simulink model "HydraTail"  (R2014b)
settings: Solver=ode3  StartTime=0.0  StopTime=inf  FixedStep=tModel  RelTol=1e-3
undefined symbols (not defined in the file or in its folder): baseGRatio, baseoffset, gcbh, rmidispblock, tipGRatio, tipoffset, tModel
libraries: legoev3lib x12, EV3Fcns x4, simulink x1
settings Model: DataDictionary=HydraTail.sldd  SimulationMode=external  ExtModeTrigDuration=2  Creator=pkaniara  LastModifiedBy=menkh
settings OptimizationCC: OptimizeModelRefInitCode=on  LifeSpan=1
settings DebuggingCC: UnderspecifiedInitializationDetection=Classic  MergeDetectMultiDrivingBlocksExec=none  SolverPrmCheckMsg=none
settings HardwareCC: ProdLargestAtomicInteger=Long  ProdLargestAtomicFloat=Float  ProdEndianess=LittleEndian  ProdHWDeviceType=ARM Compatible->ARM 9
settings RTWCC: SystemTargetFile=realtime.tlc  GenerateMakefile=off  TemplateMakefile=realtime.tmf  Description=Run on Target Hardware  RTWVerbose=off  ProcessScript=realtime_make_rtw_hook
settings STFCustomTargetCC: TargetLibSuffix=.a  GenerateSampleERTMain=on  ERTCustomFileBanners=on  SupportNonInlinedSFcns=off  SupportVariableSizeSignals=on  MATLABClassNameForMDSCustomization=Simulink.SoftwareTarget.ERTCustomization  GRTInterface=off  SystemTargetFile=realtime.tlc
settings ERTTargetCC: GenerateSampleERTMain=on  ParMdlRefBuildCompliant=off  CompOptLevelCompliant=off  ConcurrentExecutionCompliant=off  CombineOutputUpdateFcns=off  ERTFirstTimeCompliant=off  SupportContinuousTime=on  SupportVariableSizeSignals=on  ModelStepFunctionPrototypeControlCompliant=off  CPPClassGenCompliant=off  ExtMode=on  ExtModeMexArgs='192.168.10.103' 0 17725 30  InlinedParameterPlacement=NonHierarchical  ERTSrcFileBannerTemplate=realtime_code_template.cgt  ERTHdrFileBannerTemplate=realtime_code_template.cgt  ERTDataSrcFileTemplate=realtime_code_template.cgt  ERTDataHdrFileTemplate=realtime_code_template.cgt  ERTCustomFileTemplate=realtime_file_process.tlc

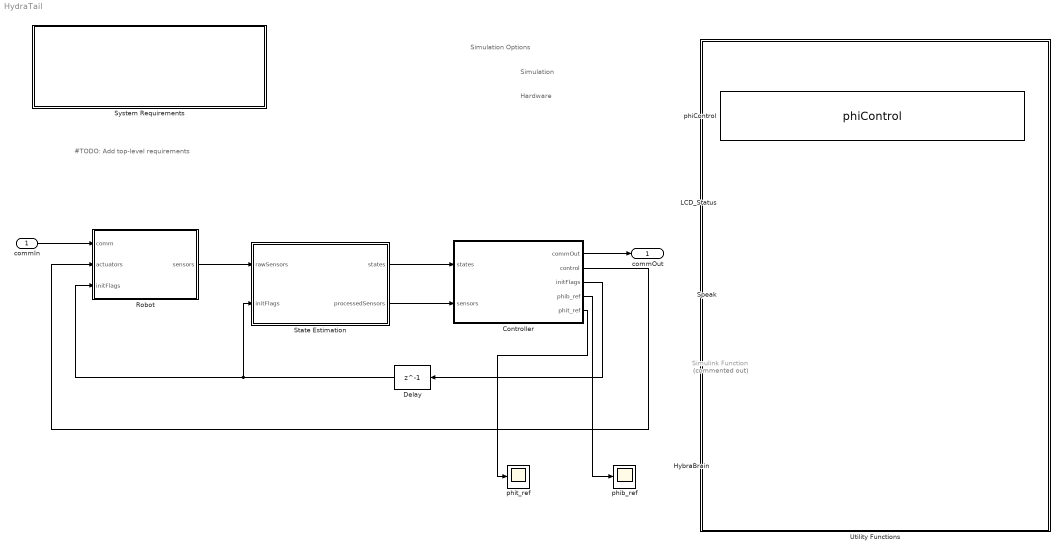
== system HydraTail ==
  note: #TODO:
      | Add top-level requirements
  note: Simulation Options
  note: Simulation
  note: Hardware
  commIn : Inport  OutDataTypeStr=Enum: Comm
  Controller : Stateflow chart  TreatAsAtomicUnit=on
  Delay : Delay  DelayLength=1  SampleTime=tModel
      settings: AttributesFormatString=Removes algebraic loop
  HybraBrain : EV3Fcns/HybraBrain
      link override 1-D Lookup Table: BreakpointsForDimension1=thetagdMod  Table=phib
      link override 1-D Lookup Table1: BreakpointsForDimension1=thetagdMod  Table=phit
  LCD_Status : EV3Fcns/LCD_Status
  Robot : Subsystem  Variant=on  VariantControl=Variant1  OverrideUsingVariant=HardwareVar
  Simulink Function : Subsystem  Commented=on  TreatAsAtomicUnit=on
  Speak : EV3Fcns/Speak
  State Estimation : Subsystem
  System Requirements : Subsystem  LoadFcn=rmidispblock('load',gcbh)  mask(System Requirements){id=SystemReq, title=System Requirements}
      mask prompts: title "Block Title"
      mask help: Lists the requirements for the current model.
      mask init:
      | id = 'SystemReq';
      | [w,h] = rmidispblock('display',gcbh);
      settings: CopyFcn=rmidispblock('create',gcbh)  DeleteFcn=rmidispblock('delete',gcbh)  ModelCloseFcn=rmidispblock('close',gcbh)  PreSaveFcn=rmidispblock('close',gcbh)  PostSaveFcn=rmidispblock('open',gcbh)  OpenFcn=rmidispblock('open',gcbh)  MoveFcn=rmidispblock('move',gcbh)
      mask Help: helpview(fullfile(docroot,'toolbox','slvnv','slvnv.map'),'systemrequirements')
      mask Display:
      | text(326/2,113-4,rmidispblock('title',gcbh),'horizontalAlignment','center','verticalAlignment','top')
      | text(w/2,h/2,'<No Requirements in System>','horizontalAlignment','center','verticalAlignment','top')
  Utility Functions : Subsystem
  phiControl : EV3Fcns/phiControl
  phib_ref : Scope
      settings: SaveName=ScopeData7
  phit_ref : Scope
      settings: SaveName=ScopeData8
  commOut : Outport  OutDataTypeStr=Enum: Comm
  wires:
  State Estimation/2(processedSensors) -> Controller/2(sensors)
  Robot/1(sensors) -> State Estimation/1(rawSensors)
  Controller/3(initFlags) -> Delay/1
  State Estimation/1(states) -> Controller/1(states)
  Delay/1 -> State Estimation/2(initFlags), Robot/3(initFlags)
  Controller/2(control) -> Robot/2(actuators)
  Controller/1(commOut) -> commOut/1
  commIn/1 -> Robot/1(comm)
  Controller/4(phib_ref) -> phib_ref/1
  Controller/5(phit_ref) -> phit_ref/1

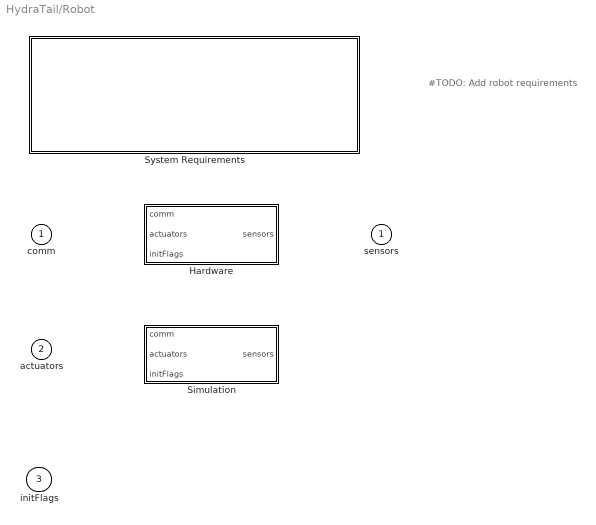
== system HydraTail/Robot ==
  note: #TODO:
      | Add robot requirements
  comm : Inport  OutDataTypeStr=Enum: Comm
  actuators : Inport  Port=2  OutDataTypeStr=Bus: ControlBus
  initFlags : Inport  Port=3  OutDataTypeStr=Bus: InitBus
  Hardware : Subsystem  VariantControl=HardwareVar
  Simulation : Subsystem  VariantControl=SimulationVar
  System Requirements : Subsystem  LoadFcn=rmidispblock('load',gcbh)  VariantControl=Variant  mask(System Requirements){id=SystemReq, title=System Requirements}
      mask prompts: title "Block Title"
      mask help: Lists the requirements for the current model.
      mask init:
      | id = 'SystemReq';
      | [w,h] = rmidispblock('display',gcbh);
      settings: CopyFcn=rmidispblock('create',gcbh)  DeleteFcn=rmidispblock('delete',gcbh)  ModelCloseFcn=rmidispblock('close',gcbh)  PreSaveFcn=rmidispblock('close',gcbh)  PostSaveFcn=rmidispblock('open',gcbh)  OpenFcn=rmidispblock('open',gcbh)  MoveFcn=rmidispblock('move',gcbh)
      mask Help: helpview(fullfile(docroot,'toolbox','slvnv','slvnv.map'),'systemrequirements')
      mask Display:
      | text(326/2,113-4,rmidispblock('title',gcbh),'horizontalAlignment','center','verticalAlignment','top')
      | text(w/2,h/2,'<No Requirements in System>','horizontalAlignment','center','verticalAlignment','top')
  sensors : Outport  OutDataTypeStr=Bus: Sensors_Bus

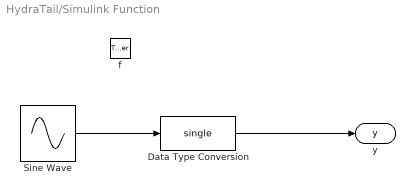
== system HydraTail/Simulink Function ==
  f : TriggerPort  TriggerType=function-call  IsSimulinkFunction=on  FunctionName=wave
  Data Type Conversion : DataTypeConversion  OutDataTypeStr=single
  Sine Wave : Sin  Amplitude=360
  y : ArgOut  DisableCoverage=on  OutDataTypeStr=single  ArgumentName=y
  wires:
  Sine Wave/1 -> Data Type Conversion/1
  Data Type Conversion/1 -> y/1

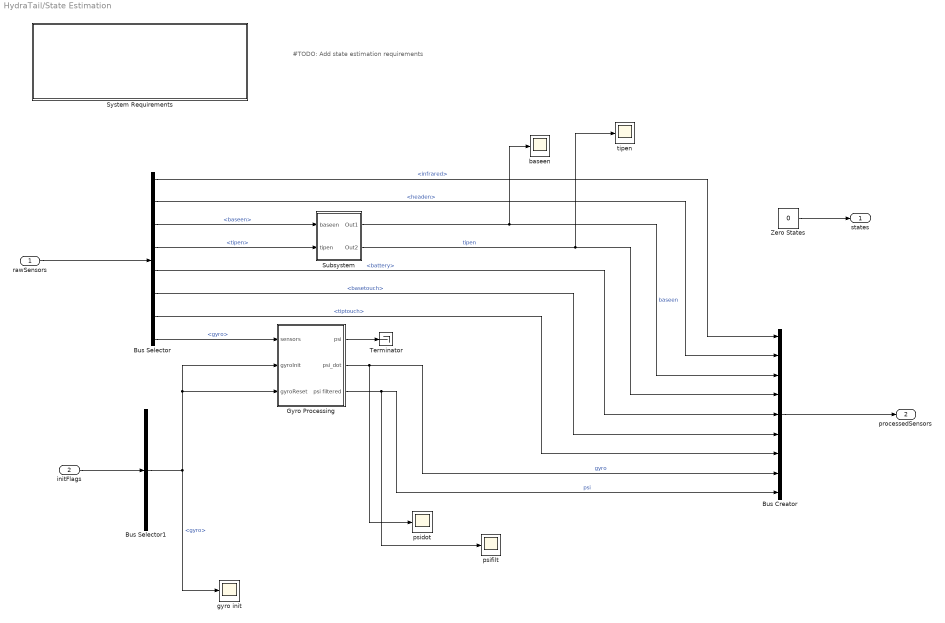
== system HydraTail/State Estimation ==
  note: #TODO:
      | Add state estimation requirements
  rawSensors : Inport  OutDataTypeStr=Bus: Sensors_Bus
  initFlags : Inport  Port=2  OutDataTypeStr=Bus: InitBus
  Bus Creator : BusCreator  Inputs=9  OutDataTypeStr=Bus: PSensors_Bus
  Bus Selector : BusSelector  OutputSignals=infrared,headen,baseen,tipen,battery,basetouch,tiptouch,gyro
  Bus Selector1 : BusSelector  OutputSignals=gyro
  Gyro Processing : Subsystem
  Subsystem : Subsystem
  System Requirements : Subsystem  LoadFcn=rmidispblock('load',gcbh)  mask(System Requirements){id=SystemReq, title=System Requirements}
      mask prompts: title "Block Title"
      mask help: Lists the requirements for the current model.
      mask init:
      | id = 'SystemReq';
      | [w,h] = rmidispblock('display',gcbh);
      settings: CopyFcn=rmidispblock('create',gcbh)  DeleteFcn=rmidispblock('delete',gcbh)  ModelCloseFcn=rmidispblock('close',gcbh)  PreSaveFcn=rmidispblock('close',gcbh)  PostSaveFcn=rmidispblock('open',gcbh)  OpenFcn=rmidispblock('open',gcbh)  MoveFcn=rmidispblock('move',gcbh)
      mask Help: helpview(fullfile(docroot,'toolbox','slvnv','slvnv.map'),'systemrequirements')
      mask Display:
      | text(326/2,113-4,rmidispblock('title',gcbh),'horizontalAlignment','center','verticalAlignment','top')
      | text(w/2,h/2,'<No Requirements in System>','horizontalAlignment','center','verticalAlignment','top')
  Terminator : Terminator
  Zero States : Constant  Value=0  OutDataTypeStr=Bus: Balancer_States_Bus  SampleTime=tModel
  baseen : Scope
      settings: YMin=107  YMax=109
  gyro init : Scope
      settings: YMin=-1  YMax=1  SaveName=ScopeData6
  psidot : Scope
      settings: YMax=4  SaveName=ScopeData2
  psifilt : Scope
      settings: YMax=10  SaveName=ScopeData3
  tipen : Scope
  states : Outport  OutDataTypeStr=Bus: Balancer_States_Bus
  processedSensors : Outport  Port=2  OutDataTypeStr=Bus: PSensors_Bus
  wires:
  Zero States/1 -> states/1
  rawSensors/1 -> Bus Selector/1
  Bus Selector/6 -> Bus Creator/6  "<basetouch>"
  Bus Selector/5 -> Bus Creator/5  "<battery>"
  Bus Creator/1 -> processedSensors/1
  Bus Selector/7 -> Bus Creator/7  "<tiptouch>"
  Bus Selector/3 -> Subsystem/1(baseen)  "<baseen>"
  Bus Selector/4 -> Subsystem/2(tipen)  "<tipen>"
  Subsystem/1(Out1) -> baseen/1, Bus Creator/3  "baseen"
  Subsystem/2(Out2) -> tipen/1, Bus Creator/4  "tipen"
  initFlags/1 -> Bus Selector1/1
  Bus Selector/8 -> Gyro Processing/1(sensors)  "<gyro>"
  Gyro Processing/3(psi filtered) -> Bus Creator/9, psifilt/1  "psi"
  Bus Selector1/1 -> Gyro Processing/3(gyroReset), Gyro Processing/2(gyroInit), gyro init/1  "<gyro>"
  Gyro Processing/2(psi_dot) -> Bus Creator/8, psidot/1  "gyro"
  Gyro Processing/1(psi) -> Terminator/1
  Bus Selector/1 -> Bus Creator/1  "<infrared>"
  Bus Selector/2 -> Bus Creator/2  "<headen>"

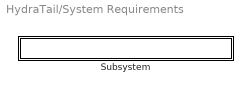
== system HydraTail/System Requirements ==
  Subsystem : Subsystem  mask{label=0, index=1}
      mask init:
      | label = rmidispblock('label',index);
      settings: OpenFcn=rmidispblock('openReq',gcbh);
      mask Display: text(0,0,label,'horizontalAlignment','left','verticalAlignment','bottom')

== system HydraTail/Utility Functions ==

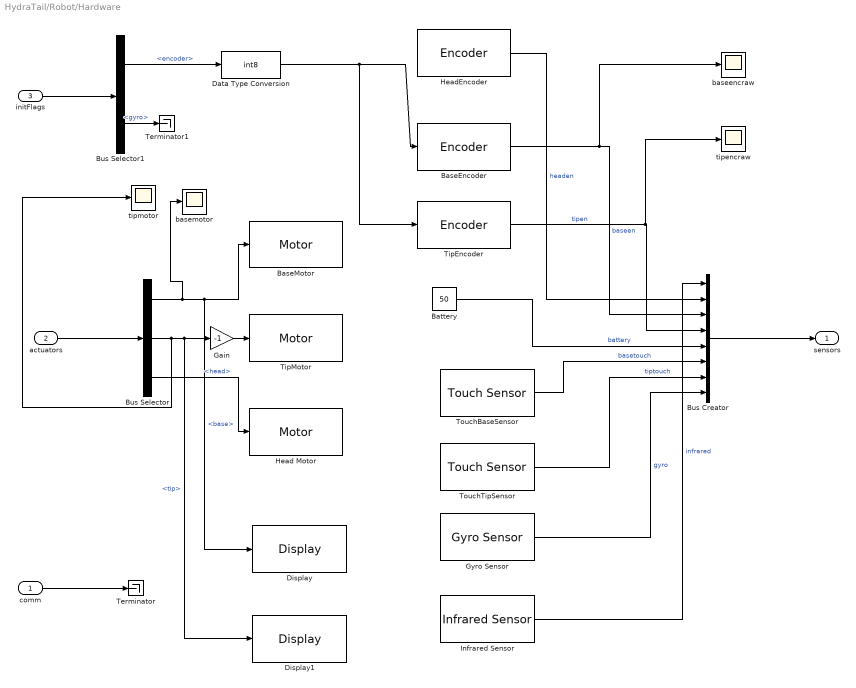
== system HydraTail/Robot/Hardware ==
  comm : Inport
  actuators : Inport  Port=2
  initFlags : Inport  Port=3  OutDataTypeStr=Bus: InitBus
  BaseEncoder : legoev3lib/Encoder  portNumber=B  opMode=Reset by external signal  sampleTime=tModel
  BaseMotor : legoev3lib/Motor  sportNumber=B  sstopAction=Brake
  Battery : Constant  Value=50  OutDataTypeStr=uint8  SampleTime=tModel
  Bus Creator : BusCreator  Inputs=8  OutDataTypeStr=Bus: Sensors_Bus
  Bus Selector : BusSelector  OutputSignals=base,tip,head
  Bus Selector1 : BusSelector  OutputSignals=encoder,gyro
  Data Type Conversion : DataTypeConversion  OutDataTypeStr=int8
  Display : legoev3lib/Display  slcdStr=Base  slcdLine=1  slcdFormat=Decimal
  Display1 : legoev3lib/Display  slcdStr=Tip  slcdLine=2  slcdFormat=Decimal
  Gain : Gain  Gain=-1
  Gyro Sensor : legoev3lib/Gyro Sensor  portNumber=1  sampleTime=tModel
  Head Motor : legoev3lib/Motor  sportNumber=C  sstopAction=Brake
  HeadEncoder : legoev3lib/Encoder  portNumber=C  opMode=No reset  sampleTime=tModel
  Infrared Sensor : legoev3lib/Infrared Sensor  portNumber=4  channelNumber=2  sampleTime=tModel
  Terminator : Terminator
  Terminator1 : Terminator
  TipEncoder : legoev3lib/Encoder  portNumber=A  opMode=Reset by external signal  sampleTime=tModel
  TipMotor : legoev3lib/Motor  sportNumber=A  sstopAction=Brake
  TouchBaseSensor : legoev3lib/Touch Sensor  portNumber=3  sampleTime=tModel
  TouchTipSensor : legoev3lib/Touch Sensor  portNumber=2  sampleTime=tModel
  baseencraw : Scope
      settings: YMin=-368  YMax=-367  SaveName=ScopeData9
  basemotor : Scope
      settings: SaveName=ScopeData4
  tipencraw : Scope
      settings: YMin=-1798  YMax=-1796  SaveName=ScopeData10
  tipmotor : Scope
      settings: SaveName=ScopeData5
  sensors : Outport  OutDataTypeStr=Bus: Sensors_Bus
  wires:
  comm/1 -> Terminator/1
  Bus Selector/1 -> basemotor/1, Display/1, BaseMotor/1  "<base>"
  actuators/1 -> Bus Selector/1
  Bus Selector/2 -> tipmotor/1, Display1/1, Gain/1  "<tip>"
  Bus Selector/3 -> Head Motor/1  "<head>"
  Bus Creator/1 -> sensors/1
  TipEncoder/1 -> tipencraw/1, Bus Creator/4  "tipen"
  BaseEncoder/1 -> baseencraw/1, Bus Creator/3  "baseen"
  Battery/1 -> Bus Creator/5  "battery"
  HeadEncoder/1 -> Bus Creator/2  "headen"
  TouchBaseSensor/1 -> Bus Creator/6  "basetouch"
  TouchTipSensor/1 -> Bus Creator/7  "tiptouch"
  Gyro Sensor/1 -> Bus Creator/8  "gyro"
  initFlags/1 -> Bus Selector1/1
  Bus Selector1/1 -> Data Type Conversion/1  "<encoder>"
  Bus Selector1/2 -> Terminator1/1  "<gyro>"
  Data Type Conversion/1 -> TipEncoder/1, BaseEncoder/1
  Gain/1 -> TipMotor/1
  Infrared Sensor/1 -> Bus Creator/1  "infrared"

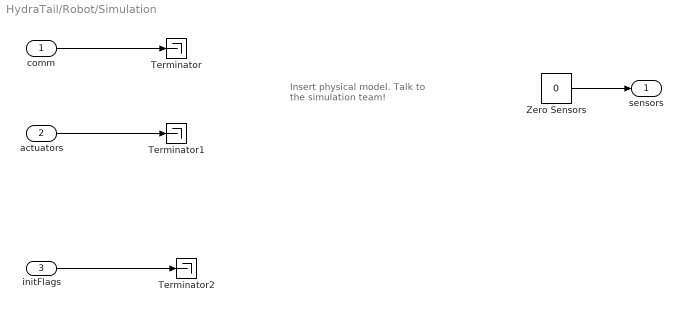
== system HydraTail/Robot/Simulation ==
  note: Insert physical model.
      | Talk to the simulation team!
  comm : Inport
  actuators : Inport  Port=2
  initFlags : Inport  Port=3  OutDataTypeStr=Bus: InitBus
  Terminator : Terminator
  Terminator1 : Terminator
  Terminator2 : Terminator
  Zero Sensors : Constant  Value=0  OutDataTypeStr=Bus: SensorsBus
  sensors : Outport
  wires:
  Zero Sensors/1 -> sensors/1
  actuators/1 -> Terminator1/1
  comm/1 -> Terminator/1
  initFlags/1 -> Terminator2/1

== system HydraTail/Robot/System Requirements ==
  Subsystem : Subsystem  mask{label=0, index=1}
      mask init:
      | label = rmidispblock('label',index);
      settings: OpenFcn=rmidispblock('openReq',gcbh);
      mask Display: text(0,0,label,'horizontalAlignment','left','verticalAlignment','bottom')

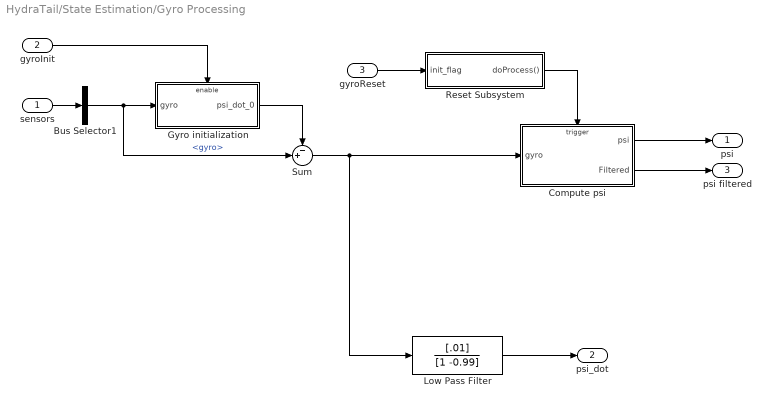
== system HydraTail/State Estimation/Gyro Processing ==
  sensors : Inport
  gyroInit : Inport  Port=2
  gyroReset : Inport  Port=3
  Bus Selector1 : BusSelector  OutputSignals=gyro
  Compute psi : Subsystem
  Gyro initialization : Subsystem  TreatAsAtomicUnit=on
  Low Pass Filter : DiscreteFilter  Numerator=[.01]  Denominator=[1 -0.99]
  Reset Subsystem : Stateflow chart  TreatAsAtomicUnit=on
  Sum : Sum  Inputs=-+|
  psi : Outport
  psi_dot : Outport  Port=2
  psi filtered : Outport  Port=3
  wires:
  Compute psi/2(Filtered) -> psi filtered/1
  Reset Subsystem/1(doProcess()) -> Compute psi/Trigger
  gyroReset/1 -> Reset Subsystem/1(init_flag)
  Bus Selector1/1 -> Sum/2, Gyro initialization/1(gyro)  "<gyro>"
  Gyro initialization/1(psi_dot_0) -> Sum/1
  Sum/1 -> Low Pass Filter/1, Compute psi/1(gyro)
  Compute psi/1(psi) -> psi/1
  sensors/1 -> Bus Selector1/1
  gyroInit/1 -> Gyro initialization/Enable
  Low Pass Filter/1 -> psi_dot/1

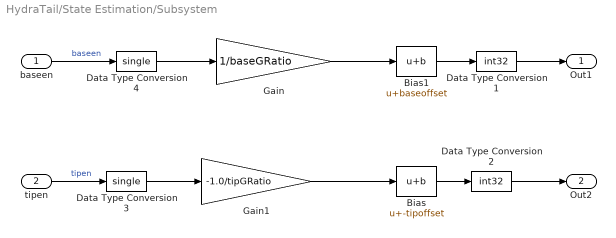
== system HydraTail/State Estimation/Subsystem ==
  baseen : Inport
  tipen : Inport  Port=2
  Bias : Bias  Bias=-tipoffset
  Bias1 : Bias  Bias=baseoffset
  Data Type Conversion1 : DataTypeConversion  OutDataTypeStr=int32
  Data Type Conversion2 : DataTypeConversion  OutDataTypeStr=int32
  Data Type Conversion3 : DataTypeConversion  OutDataTypeStr=single
  Data Type Conversion4 : DataTypeConversion  OutDataTypeStr=single
  Gain : Gain  Gain=1/baseGRatio  ParamDataTypeStr=single  OutDataTypeStr=single
  Gain1 : Gain  Gain=-1.0/tipGRatio  OutDataTypeStr=single
  Out1 : Outport
  Out2 : Outport  Port=2
  wires:
  tipen/1 -> Data Type Conversion3/1  "tipen"
  baseen/1 -> Data Type Conversion4/1  "baseen"
  Gain/1 -> Bias1/1
  Gain1/1 -> Bias/1
  Bias/1 -> Data Type Conversion2/1
  Bias1/1 -> Data Type Conversion1/1
  Data Type Conversion1/1 -> Out1/1
  Data Type Conversion2/1 -> Out2/1
  Data Type Conversion3/1 -> Gain1/1
  Data Type Conversion4/1 -> Gain/1

== system HydraTail/State Estimation/System Requirements ==
  Subsystem : Subsystem  mask{label=0, index=1}
      mask init:
      | label = rmidispblock('label',index);
      settings: OpenFcn=rmidispblock('openReq',gcbh);
      mask Display: text(0,0,label,'horizontalAlignment','left','verticalAlignment','bottom')

== system HydraTail/System Requirements/Subsystem ==

== system HydraTail/Robot/System Requirements/Subsystem ==

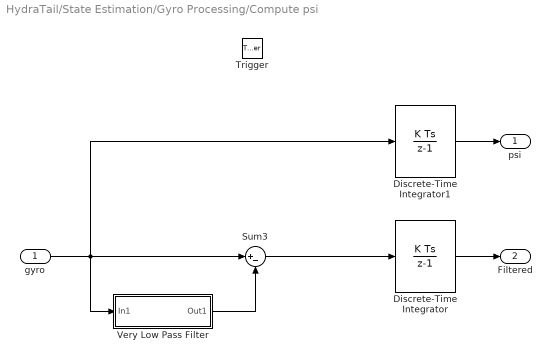
== system HydraTail/State Estimation/Gyro Processing/Compute psi ==
  gyro : Inport
  Trigger : TriggerPort  TriggerType=function-call  StatesWhenEnabling=reset  PortDimensions=1
  Discrete-Time Integrator : DiscreteIntegrator  SampleTime=-1
  Discrete-Time Integrator1 : DiscreteIntegrator  SampleTime=-1
  Sum3 : Sum  Inputs=|+-
  Very Low Pass Filter : Subsystem
  psi : Outport  InitialOutput=0
  Filtered : Outport  Port=2  InitialOutput=0
  wires:
  Discrete-Time Integrator/1 -> Filtered/1
  Discrete-Time Integrator1/1 -> psi/1
  Sum3/1 -> Discrete-Time Integrator/1
  Very Low Pass Filter/1(Out1) -> Sum3/2
  gyro/1 -> Very Low Pass Filter/1(In1), Sum3/1, Discrete-Time Integrator1/1

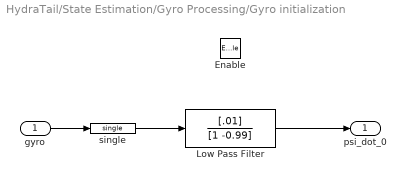
== system HydraTail/State Estimation/Gyro Processing/Gyro initialization ==
  gyro : Inport
  Enable : EnablePort  StatesWhenEnabling=reset
  Low Pass Filter : DiscreteFilter  Numerator=[.01]  Denominator=[1 -0.99]
  single : DataTypeConversion  OutDataTypeStr=single
  psi_dot_0 : Outport  InitialOutput=0
  wires:
  Low Pass Filter/1 -> psi_dot_0/1
  gyro/1 -> single/1
  single/1 -> Low Pass Filter/1

== system HydraTail/State Estimation/System Requirements/Subsystem ==

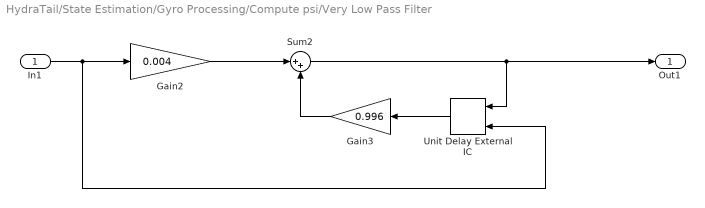
== system HydraTail/State Estimation/Gyro Processing/Compute psi/Very Low Pass Filter ==
  In1 : Inport
  Gain2 : Gain  Gain=0.004
  Gain3 : Gain  Gain=0.996
  Sum2 : Sum  Inputs=|++
  Unit Delay External IC : simulink/Additional Math & Discrete/Additional Discrete/Unit Delay External IC  tsamp=-1
  Out1 : Outport
  wires:
  Gain3/1 -> Sum2/2
  Sum2/1 -> Out1/1, Unit Delay External IC/1
  Gain2/1 -> Sum2/1
  Unit Delay External IC/1 -> Gain3/1
  In1/1 -> Gain2/1, Unit Delay External IC/2

== stateflow chart HydraTail/State Estimation/Gyro Processing/Reset Subsystem ==
  state CheckForReset
    bind: doProcess;
    entry: doProcess;
    during: doProcess;
  (default) -> CheckForReset
  CheckForReset -> CheckForReset : [init_flag == 1]
  data: init_flag input
  events: doProcess output FUNCTION_CALL_EVENT

== stateflow chart HydraTail/Controller ==
  state HeadMotion [parallel]
    en,du:
    settings: executionOrder=4
    state LookForward
      en,du:
      %do nothing
    state LookAtSpehro1
    state LookAtSpehro2
    LookForward -> LookAtSpehro1 : after(10,sec)
    LookAtSpehro1 -> LookAtSpehro2 : after(10,sec)
  state initBuses [function]
    (default) -> (junction 186) : % Control bus
        | {
        | control.tip = int8(0);
        | control.base = int8(0);
        | control.head = int8(0);
        | }
    (junction 186) -> (junction 187) : % Initialization flags
        | {
        | initFlags.encoder = false;
        | initFlags.gyro = false;
        | }
  state BaseTouchControl [parallel]
    en,du:
    settings: executionOrder=2
    state AntiClockwise
      en,du:
      control.base = base;
    state AntiClockwiseInit
      en,du:
      control.base = base;
    state NOP
      en,du:
      control.base = int8(0);
    state Clockwise
      en,du:
      control.base = base;
    state ClockwiseInit
      en,du:
      control.base = base;
    BaseTouchControl.AntiClockwise -> BaseTouchControl.NOP [order 1] : [sensors.basetouch ==1 ]{edgebase=int8(-1)}
    BaseTouchControl.AntiClockwiseInit -> BaseTouchControl.AntiClockwise [order 1] : after(1,sec)
    (default) -> BaseTouchControl.NOP
    BaseTouchControl.AntiClockwise -> BaseTouchControl.Clockwise [order 2] : [base < 0]
    BaseTouchControl.Clockwise -> BaseTouchControl.AntiClockwise [order 2] : [base > 0]
    BaseTouchControl.ClockwiseInit -> BaseTouchControl.AntiClockwise [order 2] : [base>0]
    BaseTouchControl.NOP -> BaseTouchControl.AntiClockwiseInit [order 2] : [base > 0 && edgebase > 0]
    BaseTouchControl.AntiClockwiseInit -> BaseTouchControl.Clockwise [order 2] : [base<0]
    BaseTouchControl.Clockwise -> BaseTouchControl.NOP [order 1] : [sensors.basetouch ==1 ]{edgebase= int8(1) }
    BaseTouchControl.NOP -> BaseTouchControl.ClockwiseInit [order 1] : [base < 0 && edgebase < 0]
    BaseTouchControl.ClockwiseInit -> BaseTouchControl.Clockwise [order 1] : after(1,sec)
  state TipTouchControl [parallel]
    en,du:
    settings: executionOrder=3
    state AntiClockwise
      en,du:
      control.tip = tip;
    state AntiClockwiseInit
      en,du:
      control.tip = tip;
    state NOP
      en,du:
      control.tip = int8(0);
    state Clockwise
      en,du:
      control.tip = tip;
    state ClockwiseInit
      en,du:
      control.tip = tip;
    TipTouchControl.AntiClockwise -> TipTouchControl.NOP [order 1] : [sensors.tiptouch ==1 ]{edgetip=int8(-1)}
    TipTouchControl.AntiClockwiseInit -> TipTouchControl.AntiClockwise [order 1] : after(1,sec)
    (default) -> TipTouchControl.NOP
    TipTouchControl.AntiClockwise -> TipTouchControl.Clockwise [order 2] : [tip<0]
    TipTouchControl.Clockwise -> TipTouchControl.AntiClockwise [order 3] : [tip>0]
    TipTouchControl.ClockwiseInit -> TipTouchControl.AntiClockwise [order 2] : [tip > 0]
    TipTouchControl.NOP -> TipTouchControl.AntiClockwiseInit [order 2] : [tip > 0 && edgetip > 0]
    TipTouchControl.AntiClockwiseInit -> TipTouchControl.Clockwise [order 2] : [tip < 0]
    TipTouchControl.Clockwise -> TipTouchControl.NOP [order 1] : [sensors.tiptouch ==1 ]{edgetip = int8(1) }
    TipTouchControl.Clockwise -> TipTouchControl.NOP [order 2] : [sensors.basetouch == 1 && phit_ref < single(-90)]
        | {edgetip = int8(1)}
    TipTouchControl.NOP -> TipTouchControl.ClockwiseInit [order 1] : [tip < 0 && edgetip < 0]
    TipTouchControl.ClockwiseInit -> TipTouchControl.Clockwise [order 1] : after(1,sec)
  state TailBalnce [parallel]
    en,du:
    StatusLCD(25);
    settings: executionOrder=1
    state Balance
      en:
      du:
      base = int8(phiControl(phib_ref,sensors.baseen, single(20), single(15), single(-50)));
      tip = int8(phiControl(phit_ref,sensors.tipen, single(50), single(100), single(-100)));
      state Initialization2
        en:
        StatusLCD(93);
      state Initialization4
        en:
        StatusLCD(95);
        initFlags.gyro = false;
        Speak();
      state Initialization3
        en:
        StatusLCD(94);
        initFlags.gyro = true;
        Speak();
      state Balance
        en, du:
        StatusLCD(96);
        [phib_ref, phit_ref] = HydraBrain(single(0), sensors.psi, sensors.gyro);
      state CurvePath1
        en:
        StatusLCD(97);
        %base = int8(-20);
        tip = int8(-20);
      (default) -> Initialization2
      Initialization2 -> Initialization3 : after (10,sec)
      Initialization3 -> TailBalnce.Balance.Initialization4
      TailBalnce.Balance.Initialization4 -> TailBalnce.Balance.Balance : after(2, sec)
      TailBalnce.Balance.Balance -> CurvePath1 : after(10000,sec)
    state NOPState
      en:
      StatusLCD(90);
      initBuses();
      edgebase = int8(1); %-1 bottom, 1 top
      edgetip = int8(-1); %-1 bottom, 1 top
      base = int8(0);
      tip = int8(0);
      commOut = Comm.NONE;
      phib_ref = single(59.4);
      phit_ref = single(-32.6250);
    state Initialization
      en,du:
      StatusLCD(91);
      base = int8(15);
      tip = int8(-100);
    state Initialization1
      en:
      StatusLCD(91);
      initFlags.encoder = true;
      initFlags.gyro = true;
      edgetip = int8(1);
      edgebase = int8(-1);
      StatusLCD(92);
      ex:
      initFlags.encoder = false;
      initFlags.gyro = false;
    TailBalnce.Balance -> NOPState : [sensors.infrared == uint8(5)]
    (default) -> NOPState
    NOPState -> Initialization
    Initialization -> Initialization1 : after(10,sec)
    Initialization1 -> TailBalnce.Balance
  state TailTest [parallel] [commented out]
    en,du:
    StatusLCD(25);
    state RemoteTest [commented out]
      en, du:
      n = 0;
      base = int8(phiControl(phib_ref,sensors.baseen, single(20), single(15), single(-50)));
      tip = int8(phiControl(phit_ref,sensors.tipen,single(50), single(100), single(-100)));
      %base = int8(-50);
      %tip = int8(50);
      state NOPTest [commented out]
        en:
        Speak();
        StatusLCD(200);
        %tip = int8(0);
        %base = int8(0);
      state tipup [commented out]
        en, du:
        StatusLCD(201);
        phit_ref = phit_ref - single(0.5)
        %tip = int8(-100);
      state tipdown [commented out]
        en, du:
        StatusLCD(201);
        phit_ref = phit_ref + single(0.5);
        %tip = int8(100);
      state baseup [commented out]
        en, du:
        StatusLCD(201);
        phib_ref = phib_ref + single(0.5);
        %base = int8(-50);
      state basedown [commented out]
        en, du:
        StatusLCD(204);
        phib_ref = phib_ref - single(0.5);
        %base = int8(15);
      NOPTest -> basedown [commented out] : [sensors.infrared == uint8(4)]
      NOPTest -> baseup [commented out] : [sensors.infrared == uint8(3)]
      (default) -> NOPTest [commented out]
      NOPTest -> tipdown [commented out] : [sensors.infrared == uint8(2)]
      basedown -> NOPTest [commented out] : [sensors.infrared ~= uint8(4)]
      baseup -> NOPTest [commented out] : [sensors.infrared ~= uint8(3)]
      tipdown -> NOPTest [commented out] : [sensors.infrared ~= uint8(2)]
      tipup -> NOPTest [commented out] : [sensors.infrared ~= uint8(1)]
      NOPTest -> tipup [commented out] : [sensors.infrared == uint8(1)]
    state NOPStateTest [commented out]
      en:
      initBuses();
      edgebase = int8(1); %-1 bottom, 1 top
      edgetip = int8(-1); %-1 bottom, 1 top
      base = int8(0);
      tip = int8(0);
      commOut = Comm.NONE;
      phib_ref = single(90);
      phit_ref = single(0);
      %phib_ref = single(60);
    state Initialization4 [commented out]
      en,du:
      StatusLCD(100);
      base = int8(15);
      tip = int8(-100);
    state Calibration1 [commented out]
      en:
      StatusLCD(101);
      initFlags.encoder = true;
      initFlags.gyro = true;
      edgetip = int8(1);
      edgebase = int8(-1);
      du:
      initFlags.encoder = false;
      initFlags.gyro = false;
    state TestEnd [commented out]
      en,du:
      StatusLCD(999);
      base = int8(0);
      tip = int8(0);
    (default) -> NOPStateTest [commented out]
    NOPStateTest -> TailTest.Initialization4 [commented out]
    TailTest.Initialization4 -> Calibration1 [commented out] : after(10, sec)
    Calibration1 -> RemoteTest [commented out] : after(1, sec)
    RemoteTest -> TestEnd [commented out] : [sensors.infrared == uint8(5)]
  note: #TODO
      | Add requirements to Stateflow objects
      | by right-clicking and selecting the
      | Requirements Traceability option.
  data: commOut output Enum: Comm size=1; control output Bus: ControlBus size=1; states input Bus: Balancer_States_Bus size=1; sensors input Bus: PSensors_Bus size=1; initFlags output Bus: InitBus size=1; n local double; cmd local; base local int8; tip local int8; baseoffset parameter; tipoffset parameter; data local; phib_ref output; phit_ref output size=1; edgebase local int8; edgetip local int8
